simulink model "bh_smd_MAIN_for_MASK"  (R2018b)
settings: Solver=ode45  StartTime=0.0  StopTime=10.0  RelTol=1e-7
undefined symbols (not defined in the file): c, k, m, x_init, xdot_init
settings Model: Creator=bhorton  LastModifiedBy=student
settings DebuggingCC: LibraryContextMissingDiagnostic=none
settings SFSimCC: SimUseLocalCustomCode=off
settings RTWCC: RTWUseLocalCustomCode=off
settings CodeAppCC: StateflowObjectComments=on

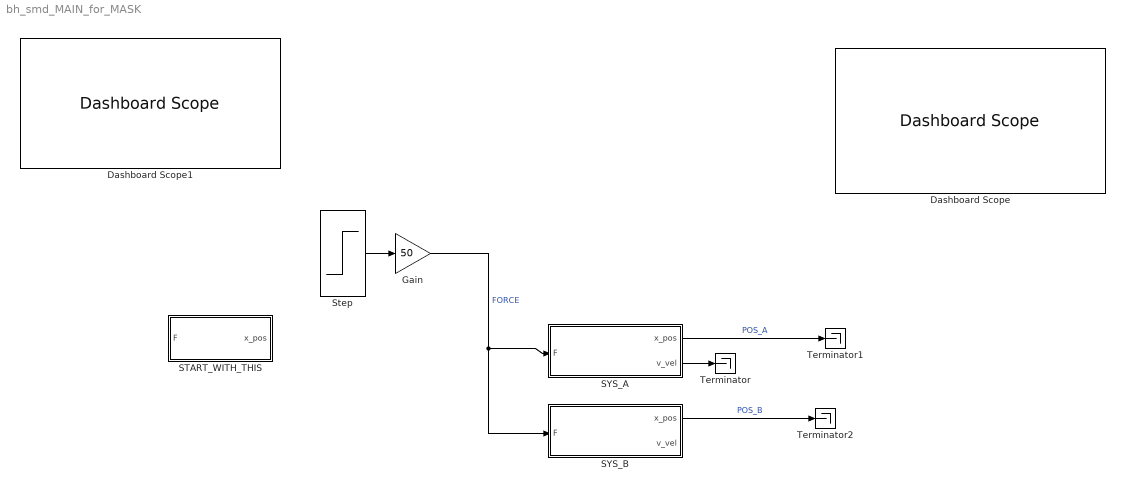
== system bh_smd_MAIN_for_MASK ==
  Dashboard Scope : DashboardScope  WebBlockId=91
  Dashboard Scope1 : DashboardScope  WebBlockId=90
  Gain : Gain  Gain=50
  START_WITH_THIS : Subsystem  mask{my_m=1, my_k=k, my_c=0.25, my_x_init=1100, my_xdot_init=0}
      mask prompts: my_m "Mass:"; my_k "Stiff:"; my_c "Damping:"; my_x_init "Initial Position:"; my_xdot_init "Initial Velocity:"
  SYS_A : Subsystem  mask{my_m=m, my_k=k, my_c=c, my_x_init=x_init, my_xdot_init=xdot_init}
      mask prompts: my_m "The MASS is"; my_k "The STIFFNESS is"; my_c "The DAMPING is"; my_x_init "the init POS is"; my_xdot_init "the init VEL is"
      mask DialogControl DescTextVar Prompt: Hello this is a Spring Mass Damper model
      mask DialogControl Container4 Prompt: Mech stuff
      mask DialogControl Container5 Prompt: Init Cond stuff
      mask Display: image('PICS_SMD.JPG');
  SYS_B : Subsystem  mask{my_m=m, my_k=k, my_c=12, my_x_init=x_init, my_xdot_init=xdot_init}
      mask prompts: my_m "The MASS is"; my_k "The STIFFNESS is"; my_c "The DAMPING is"; my_x_init "the init POS is"; my_xdot_init "the init VEL is"
      mask DialogControl DescTextVar Prompt: Hello this is a Spring Mass Damper model
      mask DialogControl Container4 Prompt: Mech stuff
      mask DialogControl Container5 Prompt: Init Cond stuff
      mask Display: image('PICS_SMD.JPG');
  Step : Step  Time=5  SampleTime=0
  Terminator : Terminator
  Terminator1 : Terminator
  Terminator2 : Terminator
  wires:
  Step/1 -> Gain/1
  Gain/1 -> SYS_B/1(F), SYS_A/1(F)  "FORCE"
  SYS_A/1(x_pos) -> Terminator1/1  "POS_A"
  SYS_A/2(v_vel) -> Terminator/1
  SYS_B/1(x_pos) -> Terminator2/1  "POS_B"

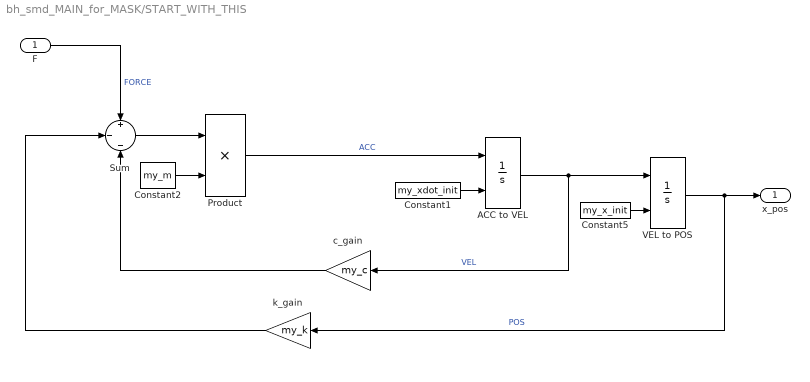
== system bh_smd_MAIN_for_MASK/START_WITH_THIS ==
  F : Inport
  ACC to VEL : Integrator  InitialConditionSource=external
  Constant1 : Constant  Value=my_xdot_init
  Constant2 : Constant  Value=my_m
  Constant5 : Constant  Value=my_x_init
  Product : Product
  Sum : Sum  Inputs=+|-|-
  VEL to POS : Integrator  InitialConditionSource=external
  c_gain : Gain  Gain=my_c
  k_gain : Gain  Gain=my_k
  x_pos : Outport
  wires:
  k_gain/1 -> Sum/2
  Sum/1 -> Product/1
  Constant1/1 -> ACC to VEL/2
  c_gain/1 -> Sum/3
  F/1 -> Sum/1  "FORCE"
  Constant5/1 -> VEL to POS/2
  VEL to POS/1 -> x_pos/1, k_gain/1  "POS"
  Product/1 -> ACC to VEL/1  "ACC"
  ACC to VEL/1 -> c_gain/1, VEL to POS/1  "VEL"
  Constant2/1 -> Product/2

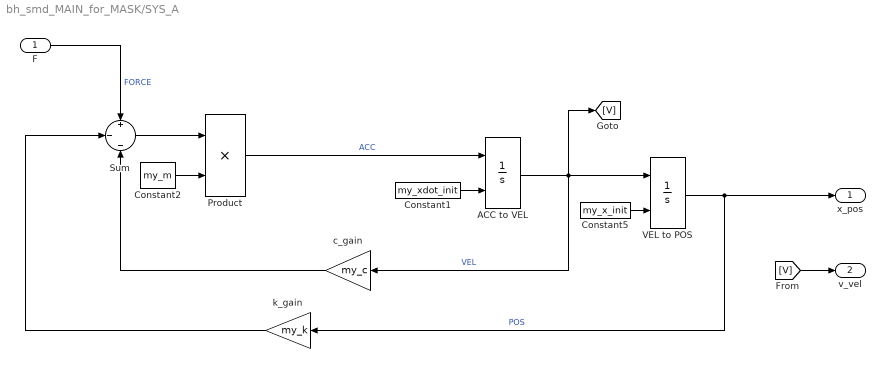
== system bh_smd_MAIN_for_MASK/SYS_A ==
  F : Inport
  ACC to VEL : Integrator  InitialConditionSource=external
  Constant1 : Constant  Value=my_xdot_init
  Constant2 : Constant  Value=my_m
  Constant5 : Constant  Value=my_x_init
  Product : Product
  Sum : Sum  Inputs=+|-|-
  VEL to POS : Integrator  InitialConditionSource=external
  c_gain : Gain  Gain=my_c
  k_gain : Gain  Gain=my_k
  x_pos : Outport
  v_vel : Outport  Port=2
  wires:
  k_gain/1 -> Sum/2
  Sum/1 -> Product/1
  Constant1/1 -> ACC to VEL/2
  c_gain/1 -> Sum/3
  F/1 -> Sum/1  "FORCE"
  Constant5/1 -> VEL to POS/2
  VEL to POS/1 -> x_pos/1, k_gain/1  "POS"
  Product/1 -> ACC to VEL/1  "ACC"
  ACC to VEL/1 -> [V], c_gain/1, VEL to POS/1  "VEL"
  Constant2/1 -> Product/2
  [V] -> v_vel/1

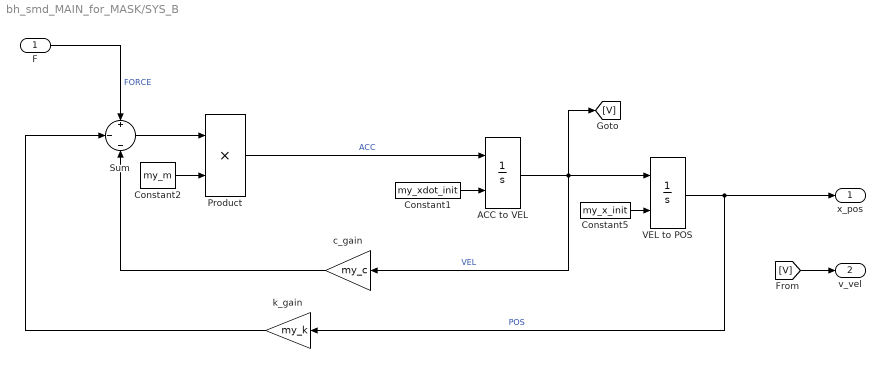
== system bh_smd_MAIN_for_MASK/SYS_B ==
  F : Inport
  ACC to VEL : Integrator  InitialConditionSource=external
  Constant1 : Constant  Value=my_xdot_init
  Constant2 : Constant  Value=my_m
  Constant5 : Constant  Value=my_x_init
  Product : Product
  Sum : Sum  Inputs=+|-|-
  VEL to POS : Integrator  InitialConditionSource=external
  c_gain : Gain  Gain=my_c
  k_gain : Gain  Gain=my_k
  x_pos : Outport
  v_vel : Outport  Port=2
  wires:
  k_gain/1 -> Sum/2
  Sum/1 -> Product/1
  Constant1/1 -> ACC to VEL/2
  c_gain/1 -> Sum/3
  F/1 -> Sum/1  "FORCE"
  Constant5/1 -> VEL to POS/2
  VEL to POS/1 -> x_pos/1, k_gain/1  "POS"
  Product/1 -> ACC to VEL/1  "ACC"
  ACC to VEL/1 -> [V], c_gain/1, VEL to POS/1  "VEL"
  Constant2/1 -> Product/2
  [V] -> v_vel/1
